simulink model "bolide_modele_simul"  (R2023b)
settings: Solver=VariableStepAuto  StartTime=0.0  StopTime=10.0  RelTol=1e-3
model workspace (MATLAB code in the model file):
  | %% Paramètres nominaux du système
  | % Masses
  | mw=0.1;
  | mb=1;
  | M=1.2;
  | 
  | % Distances
  | rho=0.07;
  | l=0.02;
  | d=0.015; % distance A-C
  | 
  | % Electriques
  | L=0.05;
  | R=1e6;
  | % r;
  | 
  | % Couples
  | k=2.63e4;
  | alpha=34.6;
  | beta=2.06e5;
  | 
  | % Moments inertie
  | Iwy=2.45e-4;
  | Ipsi=1.53e-2;
  | 
  | %% Position d'équilibre
  | ubar = 0.3; % m/s
  | psibar = 0;
  | vbar = 0;
  | ilbar = 0;
  | irbar = 0;
  | Ulbar = k*alpha;
  | Urbar = k*alpha;
settings Model: Creator=Jules  LastModifiedBy=Jules

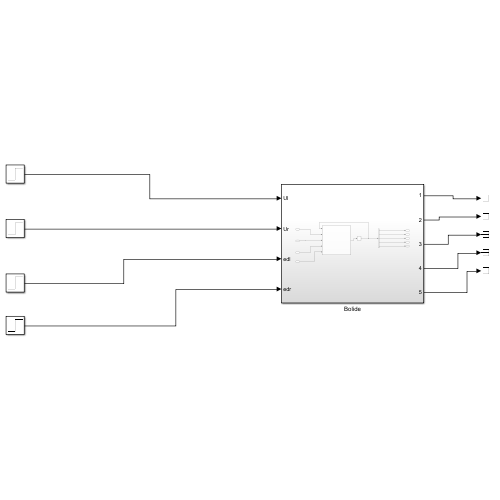
[thumbnail: Simulink's stored preview of the top-level diagram]
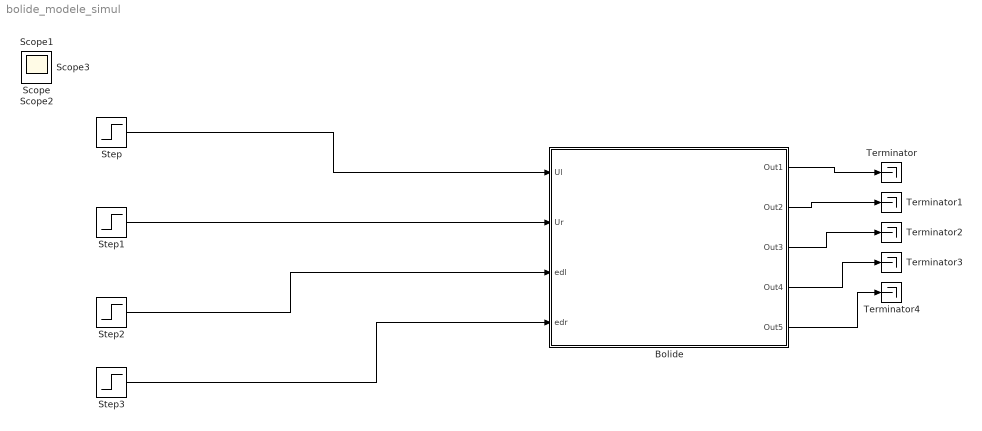
== system bolide_modele_simul ==
  Bolide : Subsystem
  Step{,1..3} (4 alike) : Step  SampleTime=0
  Terminator{,1..4} (5 alike) : Terminator
  Scope{,1..3} (4 alike) : Scope
  wires:
  Step/1 -> Bolide/1(Ul)
  Step1/1 -> Bolide/2(Ur)
  Step2/1 -> Bolide/3(edl)
  Step3/1 -> Bolide/4(edr)
  Bolide/1(Out1) -> Terminator/1
  Bolide/2(Out2) -> Terminator1/1
  Bolide/3(Out3) -> Terminator2/1
  Bolide/4(Out4) -> Terminator3/1
  Bolide/5(Out5) -> Terminator4/1

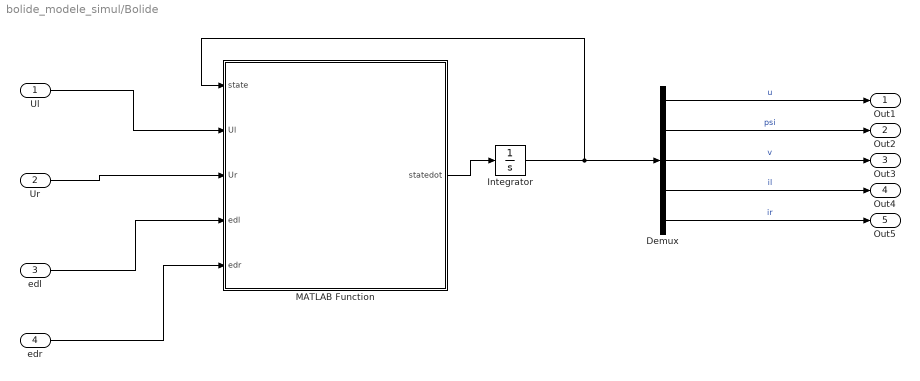
== system bolide_modele_simul/Bolide ==
  Ul : Inport
  Ur : Inport  Port=2
  edl : Inport  Port=3
  edr : Inport  Port=4
  Demux : Demux  Outputs=5
  Integrator : Integrator
  MATLAB Function : MATLAB Function  TreatAsAtomicUnit=on
  Out1 : Outport
  Out2 : Outport  Port=2
  Out3 : Outport  Port=3
  Out4 : Outport  Port=4
  Out5 : Outport  Port=5
  wires:
  edr/1 -> MATLAB Function/5(edr)
  MATLAB Function/1(statedot) -> Integrator/1
  Integrator/1 -> MATLAB Function/1(state), Demux/1
  Demux/1 -> Out1/1  "u"
  Demux/4 -> Out4/1  "il"
  Demux/5 -> Out5/1  "ir"
  Demux/2 -> Out2/1  "psi"
  Demux/3 -> Out3/1  "v"
  edl/1 -> MATLAB Function/4(edl)
  Ur/1 -> MATLAB Function/3(Ur)
  Ul/1 -> MATLAB Function/2(Ul)

== matlab function bolide_modele_simul/Bolide/MATLAB Function ==
  data: state input; statedot output; Ul input; Ur input; edl input; edr input; M parameter; rho parameter; l parameter; Iwy parameter; Ipsi parameter; d parameter; L parameter; R parameter; k parameter; mb parameter; alpha parameter; beta parameter
function statedot = fcn(state,Ul,Ur,edl,edr,M, rho, l, Iwy, Ipsi, d, L, R, k, mb, alpha, beta)
% ed est l'entrée de perturbation, != d (distance AC)
% Model parameters M,Ipsi,d,L,R,k defined in "Model Explorer/Matlab Code"

u = state(1);
psi = state(2);
v = state(3); % psidot
il = state(4); % Intensité à gauche
ir = state(5);

udot = 1/(M + 2*Iwy/rho)*(1/rho*(il + ir) - mb*d*v^2);
psidot = v;
vdot = 1/(Ipsi + mb*d^2)*(l*k/(2*rho)*(ir - il) + mb*d*u*v);
ildot = 1/L*(Ul + (beta*k^2 - R)*il - k*alpha);
irdot = 1/L*(Ur + (beta*k^2 - R)*il - k*alpha);

statedot = [udot; psidot; vdot; ildot; irdot];
